simulink model "step2"  (R2015a)
settings: Solver=ode45  StartTime=0.0  StopTime=1  RelTol=1e-3
values from neighbouring files (symbols this model uses):
  apsk32 = [R2*exp(2*pi*1i*1/12+1i*pi/12)     R2*exp(2*pi*1i*0/12+1i*pi/12)     R3*exp(2*pi*1i*1/16)     R3*exp(2*pi*1i*0/16)     R2*exp(2*pi*1i*4/12+1i*pi/12)     R2*exp(2*pi*1i*5/12+1i*pi/12)     R3*exp(2*pi*1i*6/16)     R3*exp(2*pi*1i*7/16)     R2*exp(2*pi*1i*10/12+1i*pi/12)     R2*exp(2*pi*1i*11/12+1i*pi/12)     R3*exp(2*pi*1i*14/16)     R3*exp(2*pi*1i*15/16)     R2*exp(2*pi*1i*7/12+1i*pi/12)     R2*exp( ...(+546 chars)    [DVBs2.m]    (also in DVBs2_2.m; Script.m; Test.m = apsk32*n; graphfunc.m = apsk32*n)
  Dt = 1/(SampleRate*(N_in/N_out))    [DVBs2.m]    (also in DVBs2_2.m; Script.m)
  K_BCH = 51648    [DVBs2.m]    (also in DVBs2_2.m; Script.m)
  N_in = BBHEADER + DFL    [DVBs2.m]    (also in DVBs2_2.m; Script.m)
  Poly_ampl = polyfit(Xampl_0,DPDampl_0,PolyOrder)    [step1func.m]
  Poly_phase = polyfit(Xampl_0,DPDphase_0,PolyOrder)    [step1func.m]
  roll_off = 0.25    [DVBs2.m]    (also in DVBs2_2.m; Script.m)
undefined symbols (not defined in the file or in its folder): gcbh, magnitude, rcfiltgaincompat
libraries: commfilt2 x5, commblkcod2 x4, commutil2 x3, commrflib2 x2, dsppolyfun x2, dspsigops x2, commsequence2 x2, commblkintrlv2 x2, dspstat3 x2, commdigbbndam3 x2, commchan3 x1, commrandsrc2 x1
settings Model: Creator=Study  LastModifiedBy=Наталья
settings DataIOCC: SignalLoggingSaveFormat=ModelDataLogs
settings DebuggingCC: FcnCallInpInsideContextMsg=UseLocalSettings
settings GRTTargetCC: CombineOutputUpdateFcns=off  GRTInterface=on

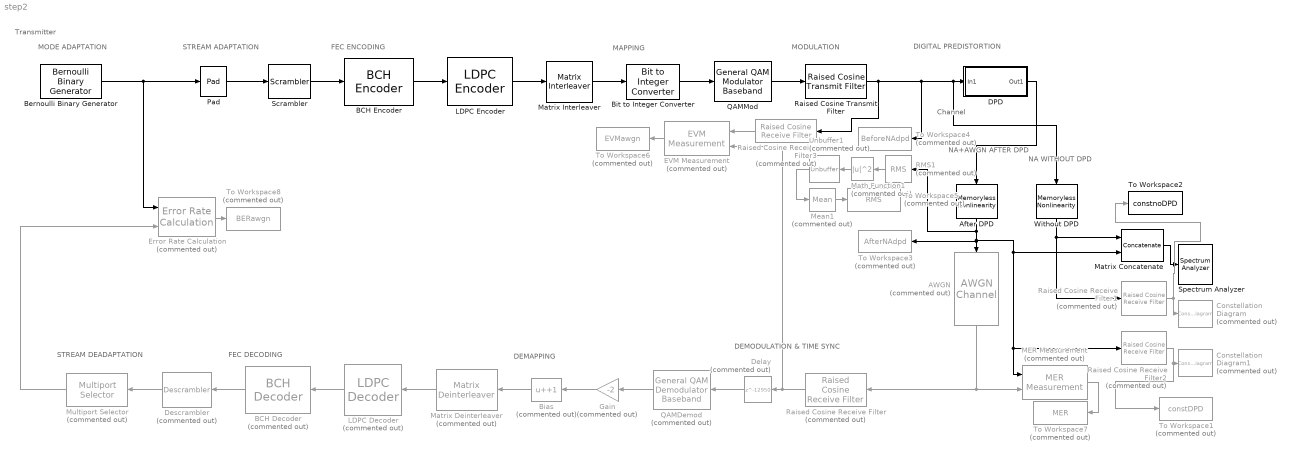
== system step2 ==
  note: DIGITAL PREDISTORTION
  note: DEMODULATION & TIME SYNC
  note: DEMAPPING
  note: FEC DECODING
  note: STREAM DEADAPTATION
  note: NA+AWGN
      | AFTER DPD
  note: Channel
  note: MODULATION
  note: MAPPING
  note: FEC ENCODING
  note: STREAM ADAPTATION
  note: MODE ADAPTATION
  note: Transmitter
  note: NA  WITHOUT
      | DPD
  AWGN : commchan3/AWGN Channel  Commented=on  InputProcessing=Columns as channels (frame based)  seed=67  noiseMode="Signal to noise ratio  (SNR)"  EbNodB=10  EsNodB=10  SNRdB=30  bitsPerSym=1  Ps=0.2036  Tsym=1  variance=1
  After DPD : commrflib2/Memoryless Nonlinearity  model_select=Saleh model  linGaindB=0  GindB=0  iip3=30  am2pm=10  LPwrLimAMPM=10  UPwrLimAMPM=inf  amam=AM_AM  ampm=AM_PM  x=[8.1081 1.5413 6.5202 -0.0718]  y=[4.6645 2.0965 10.88 -0.003]  p=0.5  GoutdB=0  vsat=1
  BCH Decoder : commblkcod2/BCH Decoder  Commented=on  n=N_BCH  k=K_BCH  specShortening=off  shortenedK=5  specGenPoly=on  genPoly=BCHGeneratorPoly  specPrimPoly=on  prPoly=BCHPrimitivePoly  specDisableGenCheck=off  specPuncture=off  punctVec=[ones(8,1); zeros(2,1)]  specErasurePort=off  showNumErr=off
  BCH Encoder : commblkcod2/BCH Encoder  n=N_BCH  k=K_BCH  specShortening=off  shortenedK=5  specGenPoly=on  genPoly=BCHGeneratorPoly  specPrimPoly=on  prPoly=BCHPrimitivePoly  specDisableGenCheck=off  specPuncture=off  punctVec=[ones(8,1); zeros(2,1)]
  Bernoulli Binary Generator : commrandsrc2/Bernoulli Binary Generator  P=0.5  seed=61  Ts=Dt  frameBased=on  sampPerFrame=N_in  orient=off  outDataType=double
  Bias : Bias  Commented=on  Bias=+1
  Bit to Integer Converter : commutil2/Bit to Integer Converter  nbits=NMOD  bitOrder=MSB first  signedOutputValues=Unsigned  outDtype=Inherit via internal rule  outDtypeSigned=Inherit via internal rule
  Constellation Diagram : ConstellationDiagram  Commented=on
  Constellation Diagram1 : ConstellationDiagram  Commented=on
  DPD : Subsystem
  Delay : Delay  Commented=on  DelayLength=12950  InitialCondition=0  InputProcessing=Columns as channels (frame based)
  Descrambler : commsequence2/Descrambler  Commented=on  M=2  poly=[1 0 0 0 0 0 0 0 0 0 0 0 0 0 1 1]  iniStaSource=Dialog Parameter  ini_sta=[1 0 0 1 0 1 0 1 0 0 0 0 0 0 0]  resetViaPort=off
  EVM Measurement : commutil2/EVM Measurement  Commented=on  normMethod=Average reference signal power  averagePower=1  peakPower=1  maxOrMinOut=off  percentileOut=off  percentileVal=95  nSym=off
  Error Rate Calculation : commsink2/Error Rate Calculation  Commented=on  N=N_in  st_delay=100  cp_mode=Entire frame  subframe=[]  PMode=Port  WsName=BERawgn  RsMode2=off  stop=off  numErr=100  maxBits=1e6
  Gain : Gain  Commented=on  Gain=-2
  LDPC Decoder : commblkcod2/LDPC Decoder  Commented=on  ParityCheckMat=H  OutputFmt=Information part  DecisionType=Hard decision  OutputDataType=double  NumIter=50  DoParityCheck=on  OutputNumIter=off  OutputFinalChecks=off
  LDPC Encoder : commblkcod2/LDPC Encoder  ParityCheckMat=H
  MER Measurement : commutil2/MER Measurement  Commented=on  maxOrMinOut=off  percentileOut=off  percentileVal=95  nSym=off
  Math Function1 : Math  Commented=on  Operator=magnitude^2  SaturateOnIntegerOverflow=on
  Matrix Concatenate : Concatenate  Mode=Multidimensional array  ConcatenateDimension=2
  Matrix Deinterleaver : commblkintrlv2/Matrix Deinterleaver  Commented=on  Nrows=Numofcols  Ncols=Numofrows
  Matrix Interleaver : commblkintrlv2/Matrix Interleaver  Nrows=Numofcols  Ncols=Numofrows
  Mean1 : dspstat3/Mean  Commented=on  run=on  reset_popup=None  directionMode=Each column  dimension=1  treatSBRowAsCol=off  roiEnable=off  roiType=Rectangles  roiPortion=Entire ROI  roiOutput=Individual statistics for each ROI  roiFlag=off  outputDataTypeStr=Inherit: Same as accumulator  outputLastDataTypeStr=Inherit: Same as accumulator  outputMin=[]  outputMax=[]  roundingMode=Floor  overflowMode=off
  Multiport Selector : dspindex/Multiport Selector  Commented=on  rowsOrCols=Rows  idxCellArray=[1:N_in]  idxErrMode=Clip Index
  Pad : dspsigops/Pad  padAlong=Columns  dimsToPad=1  valSrc=Specify via dialog  padVal=0  spec=Output size  padNumOutRowsSpecMethod=User-specified  numOutRows=K_BCH  padNumOutColsSpecMethod=User-specified  numOutCols=1  isVarDimsMode=off  padBeginning=0  padEnd=0  outSizeMode=User-specified  outSize=1  padSigAt=End  trunc_flag=None  roundingMode=Floor  overflowMode=off  truncOrWrapMode=Truncate  wrap_flag=None
  QAMDemod : commdigbbndam3/General QAM Demodulator Baseband  Commented=on  SigCon=[0.569019721201925+0.569019721201925i 0.777295394416168+0.208275673214243i 1.33112156537232+0.551368605544519i 1.4407956 -0.569019721201925+0.569019721201925i -0.777295394416168+0.208275673214243i -1.01879633906374+1.01879633906374i -1.33112156537232+0.551368605544519i 0.569019721201925-0.569019721201925i 0.777295394416168-0.208275673214244i 1.01879633906374-1.01879633906374i 1.33112156537232-0.55136860554452i -0.569019721201925-0.569019721201925i -0.777295394416168-0.208275673214243i -1.33112156537232-0.551368605544519i -1.4407956+1.76446571976559e-16i 0.208275673214243+0.777295394416168i 0.209198426912472+0.209198426912472i 0.551368605544519+1.33112156537232i 1.01879633906374+1.01879633906374i -0.208275673214243+0.777295394416168i -0.209198426912472+0.209198426912472i 8.82232859882795e-17+1.4407956i -0.551368605544519+1.33112156537232i 0.208275673214243-0.777295394416168i 0.209198426912472-0.209198426912472i -2.64669857964839e-16-1.4407956i 0.551368605544519-1.33112156537232i -0.208275673214244-0.777295394416168i -0.209198426912472-0.209198426912472i -0.55136860554452-1.33112156537232i -1.01879633906374-1.01879633906374i]  OutType=Bit  DecType=Hard decision  VarSource=Dialog  Variance=1  outDtypeBit=Inherit via internal rule  outDtype=Inherit via internal rule  roundingMode=Floor  overflowMode=Wrap  sigConstWordLen=16  accum1WordLen=32  accum1FracLen=30  prodInWordLen=32  prodInFracLen=30  prodOutWordLen=32  prodOutFracLen=30  accum2WordLen=32  accum2FracLen=30  accum3WordLen=32  accum3FracLen=30  nsiWordLen=32  nsiFracLen=30  invn0WordLen=16  invn0FracLen=8  outputWordLen=32  outputFracLen=30
  QAMMod : commdigbbndam3/General QAM Modulator Baseband  SigCon=apsk32*0.9  outDtype=double  outWordLen=16  outUDDataType=sfix(16)  outFracLenMode=Best precision  outFracLen=15
  RMS1 : dspstat3/RMS  Commented=on  run=off  reset_popup=None  InputProcessing=Columns as channels (frame based)  directionMode=Each column  dimension=1  treatSBRowAsCol=off
  Raised Cosine Receive Filter : commfilt2/Raised Cosine Receive Filter  Commented=on  filtType=Square root  N=8  filtSpan=2*(10)/2  currentFiltSpan=2*(10)/2  D=(2*(10)/2)/2  R=roll_off  sampMode=Mute  saveAsFlag=0  rateMode=Downsampling  downFactor=8  downOffset=0  framing=Enforce single-rate processing  InputProcessing=Columns as channels (frame based)  checkGain=Normalized  filterGain=rcfiltgaincompat(gcbh)  checkCoeff=off  variableName=rcRxFilt  launchFVT=off  roundingMode=Floor  overflowMode=off
  Raised Cosine Receive Filter1 : commfilt2/Raised Cosine Receive Filter  Commented=on  filtType=Square root  N=8  filtSpan=2*(10)/2  currentFiltSpan=2*(10)/2  D=(2*(10)/2)/2  R=roll_off  sampMode=Mute  saveAsFlag=0  rateMode=Downsampling  downFactor=8  downOffset=0  framing=Enforce single-rate processing  InputProcessing=Columns as channels (frame based)  checkGain=Normalized  filterGain=rcfiltgaincompat(gcbh)  checkCoeff=off  variableName=rcRxFilt1  launchFVT=off  roundingMode=Floor  overflowMode=off
  Raised Cosine Receive Filter2 : commfilt2/Raised Cosine Receive Filter  Commented=on  filtType=Square root  N=8  filtSpan=2*(10)/2  currentFiltSpan=2*(10)/2  D=(2*(10)/2)/2  R=roll_off  sampMode=Mute  saveAsFlag=0  rateMode=Downsampling  downFactor=8  downOffset=0  framing=Enforce single-rate processing  InputProcessing=Columns as channels (frame based)  checkGain=Normalized  filterGain=rcfiltgaincompat(gcbh)  checkCoeff=off  variableName=rcRxFilt2  launchFVT=off  roundingMode=Floor  overflowMode=off
  Raised Cosine Receive Filter3 : commfilt2/Raised Cosine Receive Filter  Commented=on  filtType=Square root  N=8  filtSpan=2*(10)/2  currentFiltSpan=2*(10)/2  D=(2*(10)/2)/2  R=roll_off  sampMode=Mute  saveAsFlag=0  rateMode=Downsampling  downFactor=8  downOffset=0  framing=Enforce single-rate processing  InputProcessing=Columns as channels (frame based)  checkGain=Normalized  filterGain=rcfiltgaincompat(gcbh)  checkCoeff=off  variableName=rcRxFilt3  launchFVT=off  roundingMode=Floor  overflowMode=off
  Raised Cosine Transmit Filter : commfilt2/Raised Cosine Transmit Filter  filtType=Square root  filtSpan=2*(10)/2  currentFiltSpan=2*(10)/2  D=(2*(10)/2)/2  R=roll_off  sampMode=Mute  saveAsFlag=0  N=8  framing=Enforce single-rate processing  InputProcessing=Columns as channels (frame based)  checkGain=Normalized  filterGain=rcfiltgaincompat(gcbh)  checkCoeff=off  variableName=rcTxFilt  launchFVT=off  roundingMode=Floor  overflowMode=off
  Scrambler : commsequence2/Scrambler  M=2  poly=[1 0 0 0 0 0 0 0 0 0 0 0 0 0 1 1]  iniStaSource=Dialog Parameter  ini_sta=[1 0 0 1 0 1 0 1 0 0 0 0 0 0 0]  resetViaPort=off
  Spectrum Analyzer : SpectrumAnalyzer
  To Workspace1 : ToWorkspace  Commented=on  VariableName=constDPD  SampleTime=-1
      settings: Save2DSignal=2-D array (concatenate along first dimension)
  To Workspace2 : ToWorkspace  VariableName=constnoDPD  SampleTime=-1
      settings: Save2DSignal=2-D array (concatenate along first dimension)
  To Workspace3 : ToWorkspace  Commented=on  VariableName=AfterNAdpd  SampleTime=-1
      settings: Save2DSignal=2-D array (concatenate along first dimension)
  To Workspace4 : ToWorkspace  Commented=on  VariableName=BeforeNAdpd  SampleTime=-1
      settings: Save2DSignal=2-D array (concatenate along first dimension)
  To Workspace5 : ToWorkspace  Commented=on  VariableName=RMS  SampleTime=-1
      settings: Save2DSignal=2-D array (concatenate along first dimension)
  To Workspace6 : ToWorkspace  Commented=on  VariableName=EVMawgn  SampleTime=-1
      settings: Save2DSignal=2-D array (concatenate along first dimension)
  To Workspace7 : ToWorkspace  Commented=on  VariableName=MER  SampleTime=-1
      settings: Save2DSignal=2-D array (concatenate along first dimension)
  To Workspace8 : ToWorkspace  Commented=on  VariableName=BERawgn  SampleTime=-1
      settings: Save2DSignal=2-D array (concatenate along first dimension)
  Unbuffer1 : Unbuffer  Commented=on  SampleBasedProcessing=Same as frame based
  Without DPD : commrflib2/Memoryless Nonlinearity  model_select=Saleh model  linGaindB=0  GindB=0  iip3=30  am2pm=10  LPwrLimAMPM=10  UPwrLimAMPM=inf  amam=AM_AM  ampm=AM_PM  x=[8.1081 1.5413 6.5202 -0.0718]  y=[4.6645 2.0965 10.88 -0.003]  p=0.5  GoutdB=0  vsat=1
  wires:
  Bernoulli Binary Generator/1 -> Error Rate Calculation/1, Pad/1
  Scrambler/1 -> BCH Encoder/1
  BCH Encoder/1 -> LDPC Encoder/1
  Pad/1 -> Scrambler/1
  Matrix Interleaver/1 -> Bit to Integer Converter/1
  Bit to Integer Converter/1 -> QAMMod/1
  LDPC Encoder/1 -> Matrix Interleaver/1
  QAMMod/1 -> Raised Cosine Transmit Filter/1
  QAMDemod/1 -> Gain/1
  Gain/1 -> Bias/1
  Bias/1 -> Matrix Deinterleaver/1
  Matrix Deinterleaver/1 -> LDPC Decoder/1
  LDPC Decoder/1 -> BCH Decoder/1
  BCH Decoder/1 -> Descrambler/1
  Descrambler/1 -> Multiport Selector/1
  Delay/1 -> QAMDemod/1
  Multiport Selector/1 -> Error Rate Calculation/2
  AWGN/1 -> Raised Cosine Receive Filter/1, MER Measurement/2
  Raised Cosine Receive Filter/1 -> EVM Measurement/2, Delay/1
  After DPD/1 -> RMS1/1, To Workspace3/1, AWGN/1, MER Measurement/1, Raised Cosine Receive Filter2/1, Matrix Concatenate/2
  Raised Cosine Transmit Filter/1 -> Raised Cosine Receive Filter3/1, To Workspace4/1, Without DPD/1, DPD/1(In1)
  Matrix Concatenate/1 -> Spectrum Analyzer/1
  RMS1/1 -> Math Function1/1
  Math Function1/1 -> Unbuffer1/1
  Unbuffer1/1 -> Mean1/1
  Mean1/1 -> To Workspace5/1
  Without DPD/1 -> Raised Cosine Receive Filter1/1, Matrix Concatenate/1
  Raised Cosine Receive Filter1/1 -> Constellation Diagram/1, To Workspace2/1
  Raised Cosine Receive Filter2/1 -> To Workspace1/1, Constellation Diagram1/1
  EVM Measurement/1 -> To Workspace6/1
  Raised Cosine Receive Filter3/1 -> EVM Measurement/1
  DPD/1(Out1) -> After DPD/1
  MER Measurement/1 -> To Workspace7/1
  Error Rate Calculation/1 -> To Workspace8/1

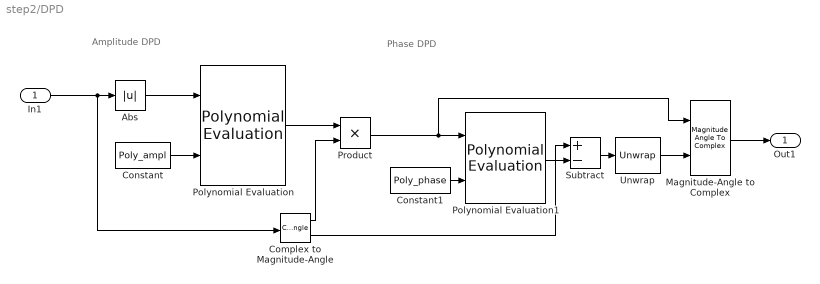
== system step2/DPD ==
  note: Phase DPD
  note: Amplitude DPD
  In1 : Inport
  Abs : Abs
  Complex to Magnitude-Angle : ComplexToMagnitudeAngle
  Constant : Constant  Value=Poly_ampl  SampleTime=-1
  Constant1 : Constant  Value=Poly_phase
  Magnitude-Angle to Complex : MagnitudeAngleToComplex
  Polynomial Evaluation : dsppolyfun/Polynomial Evaluation  useConstCoeffs=off  constCoeffs=[5 4 3 2 1]
  Polynomial Evaluation1 : dsppolyfun/Polynomial Evaluation  useConstCoeffs=off  constCoeffs=[5 4 3 2 1]
  Product : Product
  Subtract : Sum  Inputs=+-
  Unwrap : dspsigops/Unwrap  tol=pi  InputProcessing=Columns as channels (frame based)  running=off
  Out1 : Outport
  wires:
  Magnitude-Angle to Complex/1 -> Out1/1
  Unwrap/1 -> Magnitude-Angle to Complex/2
  Constant/1 -> Polynomial Evaluation/2
  Polynomial Evaluation/1 -> Product/1
  In1/1 -> Complex to Magnitude-Angle/1, Abs/1
  Abs/1 -> Polynomial Evaluation/1
  Product/1 -> Magnitude-Angle to Complex/1, Polynomial Evaluation1/1
  Constant1/1 -> Polynomial Evaluation1/2
  Polynomial Evaluation1/1 -> Subtract/2
  Complex to Magnitude-Angle/1 -> Product/2
  Subtract/1 -> Unwrap/1
  Complex to Magnitude-Angle/2 -> Subtract/1
